simulink model "random_shading"  (R2016b)
settings: Solver=VariableStepAuto  StartTime=0.0  StopTime=5  RelTol=1e-3
undefined symbols (not defined in the file or in its folder): Slope_Vdc, Ts_Power
libraries: powerlib x29, re_lib x25, simulink x2
settings Model: Creator=Gehaha  LastModifiedBy=Gehaha

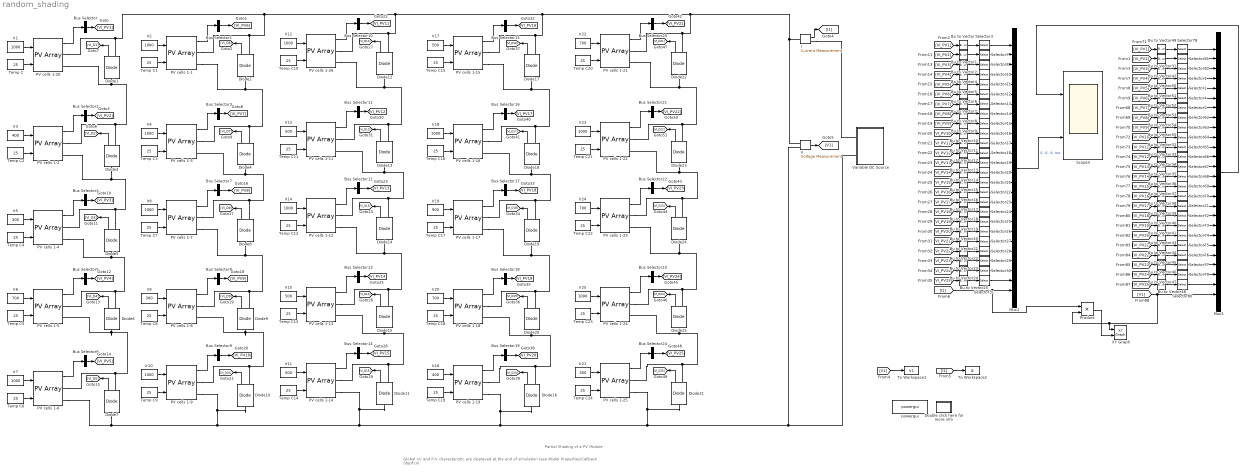
== system random_shading ==
  note: Global I-V and P-V characteristic are displayed at the end of simulation
      | (see Model Properties/Callback StopFcn)
  note: Partial Shading of a PV Module
  Bu to Vector{1..25,31..55} (50 alike) : BusToVector
  Bus Selector{,1..24} (25 alike) : BusSelector  OutputSignals=V_PV,I_PV  OutputAsBus=on
  Diode{1..25} (25 alike) : powerlib/Power Electronics/Diode  Ron=0.001  Lon=0  Vf=0.7  IC=0  UseSnubber=off  Rs=1e5*inf  Cs=inf  Measurements=on
  Double click here for more info : Subsystem
      settings: OpenFcn=showdemo(bdroot(gcb))
      mask Display: disp('?')
  I : powerlib/Measurements/Current Measurement  PhasorSimulation=off  OutputType=Complex  PSBequivalent=0
  Ir{1..2,4,7..8,10,12,14,18,23,25} (11 alike) : Constant  Value=1000
  Ir{11,13,15,17} (4 alike) : Constant  Value=500
  Ir16 : Constant  Value=400
  Ir19 : Constant  Value=900
  Ir{6,20,22,24} (4 alike) : Constant  Value=700
  Ir21 : Constant  Value=300
  Ir3 : Constant  Value=400
  Ir5 : Constant  Value=300
  Ir9 : Constant  Value=300
  Mux1 : Mux  Inputs=26
  Mux5 : Mux  Inputs=26
  PV cells 1-{1..9,11..26} (25 alike) : re_lib/Solar/PV Array  Npar=1  Nser=1  PlotType=array @ 25 deg.C & specified irradiances  S_vec="[ 1000  500  100 ]"  Temp_C_vec="[ 45 25  ]"  ModuleName=User-defined  PlotWhenSelected=off  Pm=83.2824  Ncell=60/3  Voc=37.92*20/60  Isc=8.62  Vm=30.96*20/60  Im=8.07  beta_Voc_pc=-0.33969  alpha_Isc_pc=0.063701  beta_Voc=-0.042937  alpha_Isc=0.005491  IL=8.6307  I0=1.4176e-10  nI=0.99132  Rsh=82.1161  Rs=0.098625  BAL=on  Tc=Tc  Tfilter=5e-5
  Product : Product
  Scope3 : Scope  NumInputPorts=2
  Selector{1..2,4..5,62..82} (25 alike) : Selector  InputPortWidth=2  IndexOptions=Index vector (dialog)  Indices=[1]  OutputSizes=1
  Selector{3,7..8,10..31} (25 alike) : Selector  InputPortWidth=2  IndexOptions=Index vector (dialog)  Indices=[2]  OutputSizes=1
  Temp C{,1..24} (25 alike) : Constant  Value=25
  To Workspace1 : ToWorkspace  VariableName=V1  SampleTime=1e-3
  To Workspace2 : ToWorkspace  VariableName=I1  SampleTime=1e-3
  V : powerlib/Measurements/Voltage Measurement  PhasorSimulation=off  OutputType=Complex  PSBequivalent=0
  Variable DC Source : Subsystem
  XY Graph : simulink/Sinks/XY Graph  xmin=0  xmax=70  ymin=0  ymax=2500  st=-1
  powergui : powerlib/powergui  Priority=1  SimulationMode=Continuous  SolverType=Tustin/Backward Euler (TBE)  SampleTime=Ts_Power*0 + 20e-6  frequency=60  SPID=off  DisableSnubberDevices=on  DisableRonSwitches=off  DisableVfSwitches=off  SwTol=0  DisplayEquations=off  Interpol=off  ExternalGateDelay=off  methode=off  Ts=0  FunctionMessages=off  echomessages=off  HookPort=off  EnableUseOfTLC=off  x0status=blocks  frequencyindice=0  Pbase=100e6  ErrMax=1e-4  Iterations=50  UnitsV=kV  UnitsW=MW  buscounter=0  RestoreLinks=warning  ResistiveCurrentMeasurement=off  Frange=[0:2:500]  Ylog=off  Xlog=on  ShowGrid=off  save=off  variable=ZData  structure=0  ZoomFFT=on  StartTime=0.0  cycles=1  DisplayStyle=1  fundamental=60  FreqAxis=off  MaxFrequency=1000  frequencyindicesteady=1  RmsSteady=1  display=off
  wires:
  Ir1/1 -> PV cells 1-20/1
  Temp C/1 -> PV cells 1-20/2
  I/1 -> [I1]
  V/1 -> [V1]
  Diode1/1 -> [VI_D1]
  PV cells 1-20/1 -> Bus Selector/1
  Bus Selector/1 -> [VI_PV1]
  [V1] -> To Workspace1/1
  [I1] -> To Workspace2/1
  Ir2/1 -> PV cells 1-1/1
  Temp C1/1 -> PV cells 1-1/2
  Diode2/1 -> [VI_D6]
  PV cells 1-1/1 -> Bus Selector1/1
  Bus Selector1/1 -> [VI_PV6]
  Ir3/1 -> PV cells 1-2/1
  Temp C2/1 -> PV cells 1-2/2
  Diode3/1 -> [VI_D2]
  PV cells 1-2/1 -> Bus Selector2/1
  Bus Selector2/1 -> [VI_PV2]
  Ir4/1 -> PV cells 1-3/1
  Temp C3/1 -> PV cells 1-3/2
  Diode4/1 -> [VI_D7]
  PV cells 1-3/1 -> Bus Selector3/1
  Bus Selector3/1 -> [VI_PV7]
  Ir5/1 -> PV cells 1-4/1
  Temp C4/1 -> PV cells 1-4/2
  Diode5/1 -> [VI_D3]
  PV cells 1-4/1 -> Bus Selector4/1
  Bus Selector4/1 -> [VI_PV3]
  Ir6/1 -> PV cells 1-5/1
  Temp C5/1 -> PV cells 1-5/2
  Diode6/1 -> [VI_D4]
  PV cells 1-5/1 -> Bus Selector5/1
  Bus Selector5/1 -> [VI_PV4]
  Ir7/1 -> PV cells 1-6/1
  Temp C6/1 -> PV cells 1-6/2
  Diode7/1 -> [VI_D5]
  PV cells 1-6/1 -> Bus Selector6/1
  Bus Selector6/1 -> [VI_PV5]
  Ir8/1 -> PV cells 1-7/1
  Temp C7/1 -> PV cells 1-7/2
  Diode8/1 -> [VI_D8]
  PV cells 1-7/1 -> Bus Selector7/1
  Bus Selector7/1 -> [VI_PV8]
  Ir9/1 -> PV cells 1-8/1
  Temp C8/1 -> PV cells 1-8/2
  Diode9/1 -> [VI_D9]
  PV cells 1-8/1 -> Bus Selector8/1
  Bus Selector8/1 -> [VI_PV9]
  Ir10/1 -> PV cells 1-9/1
  Temp C9/1 -> PV cells 1-9/2
  Diode10/1 -> [VI_D10]
  PV cells 1-9/1 -> Bus Selector9/1
  Bus Selector9/1 -> [VI_PV10]
  Ir12/1 -> PV cells 1-26/1
  Temp C10/1 -> PV cells 1-26/2
  Diode12/1 -> [VI_D11]
  PV cells 1-26/1 -> Bus Selector10/1
  Bus Selector10/1 -> [VI_PV11]
  Ir13/1 -> PV cells 1-11/1
  Temp C11/1 -> PV cells 1-11/2
  Diode13/1 -> [VI_D12]
  PV cells 1-11/1 -> Bus Selector11/1
  Bus Selector11/1 -> [VI_PV12]
  Ir14/1 -> PV cells 1-12/1
  Temp C12/1 -> PV cells 1-12/2
  Diode14/1 -> [VI_D13]
  PV cells 1-12/1 -> Bus Selector12/1
  Bus Selector12/1 -> [VI_PV13]
  Ir15/1 -> PV cells 1-13/1
  Temp C13/1 -> PV cells 1-13/2
  Diode15/1 -> [VI_D14]
  PV cells 1-13/1 -> Bus Selector13/1
  Bus Selector13/1 -> [VI_PV14]
  Ir11/1 -> PV cells 1-14/1
  Temp C14/1 -> PV cells 1-14/2
  Diode11/1 -> [VI_D15]
  PV cells 1-14/1 -> Bus Selector14/1
  Bus Selector14/1 -> [VI_PV15]
  Ir17/1 -> PV cells 1-15/1
  Temp C15/1 -> PV cells 1-15/2
  Diode17/1 -> [VI_D16]
  PV cells 1-15/1 -> Bus Selector15/1
  Bus Selector15/1 -> [VI_PV16]
  Ir18/1 -> PV cells 1-16/1
  Temp C16/1 -> PV cells 1-16/2
  Diode18/1 -> [VI_D17]
  PV cells 1-16/1 -> Bus Selector16/1
  Bus Selector16/1 -> [VI_PV17]
  Ir19/1 -> PV cells 1-17/1
  Temp C17/1 -> PV cells 1-17/2
  Diode19/1 -> [VI_D18]
  PV cells 1-17/1 -> Bus Selector17/1
  Bus Selector17/1 -> [VI_PV18]
  Ir20/1 -> PV cells 1-18/1
  Temp C18/1 -> PV cells 1-18/2
  Diode20/1 -> [VI_D19]
  PV cells 1-18/1 -> Bus Selector18/1
  Bus Selector18/1 -> [VI_PV19]
  Ir16/1 -> PV cells 1-19/1
  Temp C19/1 -> PV cells 1-19/2
  Diode16/1 -> [VI_D20]
  PV cells 1-19/1 -> Bus Selector19/1
  Bus Selector19/1 -> [VI_PV20]
  Ir22/1 -> PV cells 1-21/1
  Temp C20/1 -> PV cells 1-21/2
  Diode22/1 -> [VI_D21]
  PV cells 1-21/1 -> Bus Selector20/1
  Bus Selector20/1 -> [VI_PV21]
  Ir23/1 -> PV cells 1-22/1
  Temp C21/1 -> PV cells 1-22/2
  Diode23/1 -> [VI_D22]
  PV cells 1-22/1 -> Bus Selector21/1
  Bus Selector21/1 -> [VI_PV22]
  Ir24/1 -> PV cells 1-23/1
  Temp C22/1 -> PV cells 1-23/2
  Diode24/1 -> [VI_D23]
  PV cells 1-23/1 -> Bus Selector22/1
  Bus Selector22/1 -> [VI_PV23]
  Ir25/1 -> PV cells 1-24/1
  Temp C23/1 -> PV cells 1-24/2
  Diode25/1 -> [VI_D24]
  PV cells 1-24/1 -> Bus Selector23/1
  Bus Selector23/1 -> [VI_PV24]
  Ir21/1 -> PV cells 1-25/1
  Temp C24/1 -> PV cells 1-25/2
  Diode21/1 -> [VI_D25]
  PV cells 1-25/1 -> Bus Selector24/1
  Bus Selector24/1 -> [VI_PV25]
  [VI_PV1] -> Bu to Vector3/1
  Selector3/1 -> Mux1/1
  Bu to Vector3/1 -> Selector3/1
  [I1] -> Product/1, Mux1/26
  Selector7/1 -> Mux1/2
  Selector8/1 -> Mux1/3
  Selector10/1 -> Mux1/4
  Selector11/1 -> Mux1/5
  Selector12/1 -> Mux1/6
  Selector13/1 -> Mux1/7
  [VI_PV2] -> Bu to Vector1/1
  Bu to Vector1/1 -> Selector7/1
  [VI_PV3] -> Bu to Vector2/1
  Bu to Vector2/1 -> Selector8/1
  [VI_PV4] -> Bu to Vector4/1
  Bu to Vector4/1 -> Selector10/1
  [VI_PV5] -> Bu to Vector5/1
  Bu to Vector5/1 -> Selector11/1
  [VI_PV6] -> Bu to Vector6/1
  Bu to Vector6/1 -> Selector12/1
  [VI_PV7] -> Bu to Vector7/1
  Bu to Vector7/1 -> Selector13/1
  [VI_PV8] -> Bu to Vector8/1
  Bu to Vector8/1 -> Selector14/1
  Selector14/1 -> Mux1/8
  [VI_PV9] -> Bu to Vector9/1
  Bu to Vector9/1 -> Selector15/1
  Selector15/1 -> Mux1/9
  [VI_PV10] -> Bu to Vector10/1
  Bu to Vector10/1 -> Selector16/1
  Selector16/1 -> Mux1/10
  [VI_PV11] -> Bu to Vector11/1
  Bu to Vector11/1 -> Selector17/1
  Selector17/1 -> Mux1/11
  [VI_PV12] -> Bu to Vector12/1
  Bu to Vector12/1 -> Selector18/1
  Selector18/1 -> Mux1/12
  [VI_PV13] -> Bu to Vector13/1
  Bu to Vector13/1 -> Selector19/1
  Selector19/1 -> Mux1/13
  [VI_PV14] -> Bu to Vector14/1
  Bu to Vector14/1 -> Selector20/1
  Selector20/1 -> Mux1/14
  [VI_PV15] -> Bu to Vector15/1
  Bu to Vector15/1 -> Selector21/1
  Selector21/1 -> Mux1/15
  [VI_PV16] -> Bu to Vector16/1
  Bu to Vector16/1 -> Selector22/1
  Selector22/1 -> Mux1/16
  [VI_PV17] -> Bu to Vector17/1
  Bu to Vector17/1 -> Selector23/1
  Selector23/1 -> Mux1/17
  [VI_PV18] -> Bu to Vector18/1
  Bu to Vector18/1 -> Selector24/1
  Selector24/1 -> Mux1/18
  [VI_PV19] -> Bu to Vector19/1
  Bu to Vector19/1 -> Selector25/1
  Selector25/1 -> Mux1/19
  [VI_PV20] -> Bu to Vector20/1
  Bu to Vector20/1 -> Selector26/1
  Selector26/1 -> Mux1/20
  [VI_PV21] -> Bu to Vector21/1
  Bu to Vector21/1 -> Selector27/1
  Selector27/1 -> Mux1/21
  [VI_PV22] -> Bu to Vector22/1
  Bu to Vector22/1 -> Selector28/1
  Selector28/1 -> Mux1/22
  [VI_PV23] -> Bu to Vector23/1
  Bu to Vector23/1 -> Selector29/1
  Selector29/1 -> Mux1/23
  [VI_PV24] -> Bu to Vector24/1
  Bu to Vector24/1 -> Selector30/1
  Selector30/1 -> Mux1/24
  [VI_PV25] -> Bu to Vector25/1
  Bu to Vector25/1 -> Selector31/1
  Selector31/1 -> Mux1/25
  [VI_PV1] -> Bu to Vector49/1
  Selector78/1 -> Mux5/1
  Bu to Vector49/1 -> Selector78/1
  [V1] -> XY Graph/1, Product/2, Mux5/26
  Selector81/1 -> Mux5/2
  Selector82/1 -> Mux5/3
  Selector1/1 -> Mux5/4
  Selector2/1 -> Mux5/5
  Selector4/1 -> Mux5/6
  Selector5/1 -> Mux5/7
  [VI_PV2] -> Bu to Vector31/1
  Bu to Vector31/1 -> Selector81/1
  [VI_PV3] -> Bu to Vector42/1
  Bu to Vector42/1 -> Selector82/1
  [VI_PV4] -> Bu to Vector50/1
  Bu to Vector50/1 -> Selector1/1
  [VI_PV5] -> Bu to Vector51/1
  Bu to Vector51/1 -> Selector2/1
  [VI_PV6] -> Bu to Vector52/1
  Bu to Vector52/1 -> Selector4/1
  [VI_PV7] -> Bu to Vector53/1
  Bu to Vector53/1 -> Selector5/1
  [VI_PV8] -> Bu to Vector54/1
  Bu to Vector54/1 -> Selector62/1
  Selector62/1 -> Mux5/8
  [VI_PV9] -> Bu to Vector55/1
  Bu to Vector55/1 -> Selector63/1
  Selector63/1 -> Mux5/9
  [VI_PV10] -> Bu to Vector32/1
  Bu to Vector32/1 -> Selector64/1
  Selector64/1 -> Mux5/10
  [VI_PV11] -> Bu to Vector33/1
  Bu to Vector33/1 -> Selector65/1
  Selector65/1 -> Mux5/11
  [VI_PV12] -> Bu to Vector34/1
  Bu to Vector34/1 -> Selector66/1
  Selector66/1 -> Mux5/12
  [VI_PV13] -> Bu to Vector35/1
  Bu to Vector35/1 -> Selector67/1
  Selector67/1 -> Mux5/13
  [VI_PV14] -> Bu to Vector36/1
  Bu to Vector36/1 -> Selector68/1
  Selector68/1 -> Mux5/14
  [VI_PV15] -> Bu to Vector37/1
  Bu to Vector37/1 -> Selector69/1
  Selector69/1 -> Mux5/15
  [VI_PV16] -> Bu to Vector38/1
  Bu to Vector38/1 -> Selector70/1
  Selector70/1 -> Mux5/16
  [VI_PV17] -> Bu to Vector39/1
  Bu to Vector39/1 -> Selector71/1
  Selector71/1 -> Mux5/17
  [VI_PV18] -> Bu to Vector40/1
  Bu to Vector40/1 -> Selector72/1
  Selector72/1 -> Mux5/18
  [VI_PV19] -> Bu to Vector41/1
  Bu to Vector41/1 -> Selector73/1
  Selector73/1 -> Mux5/19
  [VI_PV20] -> Bu to Vector43/1
  Bu to Vector43/1 -> Selector74/1
  Selector74/1 -> Mux5/20
  [VI_PV21] -> Bu to Vector44/1
  Bu to Vector44/1 -> Selector75/1
  Selector75/1 -> Mux5/21
  [VI_PV22] -> Bu to Vector45/1
  Bu to Vector45/1 -> Selector76/1
  Selector76/1 -> Mux5/22
  [VI_PV23] -> Bu to Vector46/1
  Bu to Vector46/1 -> Selector77/1
  Selector77/1 -> Mux5/23
  [VI_PV24] -> Bu to Vector47/1
  Bu to Vector47/1 -> Selector79/1
  Selector79/1 -> Mux5/24
  [VI_PV25] -> Bu to Vector48/1
  Bu to Vector48/1 -> Selector80/1
  Selector80/1 -> Mux5/25
  Mux1/1 -> Scope3/2  "I1, I2, I3, Itot"
  Mux5/1 -> Scope3/1
  Product/1 -> XY Graph/2
  connections:
  PV cells 1-21/RConn1 -- Diode22/RConn1 -- I/LConn1 -- V/LConn1 -- PV cells 1-15/RConn1 -- Diode17/RConn1 -- PV cells 1-26/RConn1 -- Diode12/RConn1 -- Diode2/RConn1 -- PV cells 1-1/RConn1 -- Diode1/RConn1 -- PV cells 1-20/RConn1
  Diode8/RConn1 -- PV cells 1-7/RConn1 -- Diode4/LConn1 -- PV cells 1-3/RConn2
  Diode2/LConn1 -- PV cells 1-1/RConn2 -- Diode4/RConn1 -- PV cells 1-3/RConn1
  Diode1/LConn1 -- PV cells 1-20/RConn2 -- Diode3/RConn1 -- PV cells 1-2/RConn1
  Diode21/LConn1 -- PV cells 1-25/RConn2 -- V/LConn2 -- Variable DC Source/LConn2 -- PV cells 1-6/RConn2 -- Diode7/LConn1 -- Diode10/LConn1 -- PV cells 1-9/RConn2 -- Diode11/LConn1 -- PV cells 1-14/RConn2 -- Diode16/LConn1 -- PV cells 1-19/RConn2
  Diode5/RConn1 -- PV cells 1-4/RConn1 -- Diode3/LConn1 -- PV cells 1-2/RConn2
  PV cells 1-4/RConn2 -- Diode5/LConn1 -- Diode6/RConn1 -- PV cells 1-5/RConn1
  Diode7/RConn1 -- PV cells 1-6/RConn1 -- PV cells 1-5/RConn2 -- Diode6/LConn1
  PV cells 1-8/RConn1 -- Diode9/RConn1 -- PV cells 1-7/RConn2 -- Diode8/LConn1
  PV cells 1-8/RConn2 -- Diode9/LConn1 -- Diode10/RConn1 -- PV cells 1-9/RConn1
  PV cells 1-12/RConn1 -- Diode14/RConn1 -- Diode13/LConn1 -- PV cells 1-11/RConn2
  Diode12/LConn1 -- PV cells 1-26/RConn2 -- Diode13/RConn1 -- PV cells 1-11/RConn1
  Diode15/RConn1 -- PV cells 1-13/RConn1 -- Diode14/LConn1 -- PV cells 1-12/RConn2
  PV cells 1-13/RConn2 -- Diode15/LConn1 -- Diode11/RConn1 -- PV cells 1-14/RConn1
  PV cells 1-17/RConn1 -- Diode19/RConn1 -- Diode18/LConn1 -- PV cells 1-16/RConn2
  Diode17/LConn1 -- PV cells 1-15/RConn2 -- Diode18/RConn1 -- PV cells 1-16/RConn1
  Diode20/RConn1 -- PV cells 1-18/RConn1 -- Diode19/LConn1 -- PV cells 1-17/RConn2
  PV cells 1-18/RConn2 -- Diode20/LConn1 -- Diode16/RConn1 -- PV cells 1-19/RConn1
  PV cells 1-22/RConn2 -- Diode23/LConn1 -- PV cells 1-23/RConn1 -- Diode24/RConn1
  PV cells 1-22/RConn1 -- Diode23/RConn1 -- Diode22/LConn1 -- PV cells 1-21/RConn2
  PV cells 1-23/RConn2 -- Diode24/LConn1 -- Diode25/RConn1 -- PV cells 1-24/RConn1
  PV cells 1-25/RConn1 -- Diode21/RConn1 -- PV cells 1-24/RConn2 -- Diode25/LConn1
  I/RConn1 -- Variable DC Source/LConn1

== system random_shading/Double click here for more info ==

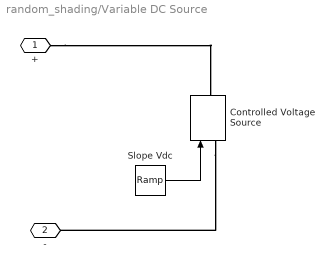
== system random_shading/Variable DC Source ==
  Controlled Voltage Source : powerlib/Electrical Sources/Controlled Voltage Source  Initialize=on  Source_Type=AC  Amplitude=0  Phase=0  Frequency=0  Measurements=None
  Slope Vdc : simulink/Sources/Ramp  slope=Slope_Vdc  start=0  X0=0
  + : PMIOPort  Port=1  Side=Left
  - : PMIOPort  Port=2  Side=Left
  wires:
  Slope Vdc/1 -> Controlled Voltage Source/1
  connections:
  Controlled Voltage Source/LConn1 -- -/RConn1
  +/RConn1 -- Controlled Voltage Source/RConn1
